simulink model "Lab3_1"  (R2016a)
settings: Solver=FixedStepDiscrete  StartTime=0.0  StopTime=10.0  RelTol=1e-3
settings Model: Creator=NoteBook  LastModifiedBy=NoteBook
settings OptimizationCC: DefaultParameterBehavior=Inlined  EnableMemcpy=off  OptimizeModelRefInitCode=on  LifeSpan=1
settings DebuggingCC: UnderspecifiedInitializationDetection=Classic  MergeDetectMultiDrivingBlocksExec=none
settings ModelReferenceCC: PropagateSignalLabelsOutOfModel=off
settings RTWCC: SystemTargetFile=ert.tlc  GenCodeOnly=on  TemplateMakefile=ert_default_tmf  GenerateReport=on  IncludeHyperlinkInReport=on  LaunchReport=on  GenerateTraceInfo=on  GenerateTraceReport=on  GenerateTraceReportSl=on  GenerateTraceReportSf=on  GenerateTraceReportEml=on
settings CodeAppCC: ForceParamTrailComments=on  IgnoreCustomStorageClasses=off  OperatorAnnotations=on  SimulinkDataObjDesc=on  SFDataObjDesc=on  MATLABFcnDesc=on  InsertBlockDesc=on  MATLABSourceComments=on
settings ERTTargetCC: GenerateSampleERTMain=on  InlinedParameterPlacement=NonHierarchical  ERTCustomFileTemplate=example_file_process.tlc

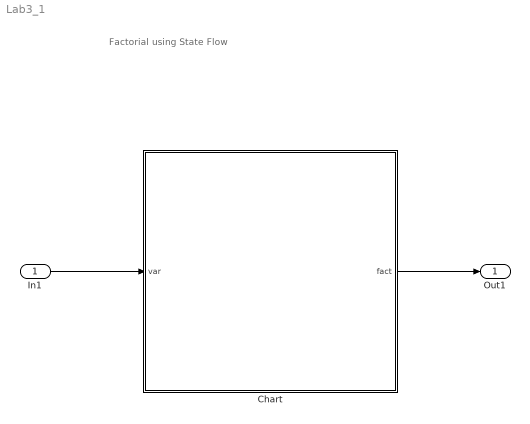
== system Lab3_1 ==
  note: Factorial using State Flow
  In1 : Inport
  Chart : Stateflow chart  TreatAsAtomicUnit=on
  Out1 : Outport
  wires:
  In1/1 -> Chart/1(var)
  Chart/1(fact) -> Out1/1

== stateflow chart Lab3_1/Chart ==
  (junction 9) -> (junction 7) [order 1] : [counter > 1]
  (junction 7) -> (junction 10) : {fact = fact * counter;}
  (default) -> (junction 8)
  (junction 8) -> (junction 9) : {counter = var ; fact = 1;}
  (junction 10) -> (junction 9) : {counter = counter - 1 ;}
  (junction 9) -> (junction 11) [order 2]
  data: var input uint8; counter local uint8 size=1; fact output int32
